simulink model "qu_sim"  (R2020a)
settings: Solver=FixedStepAuto  StartTime=0.0  StopTime=500  RelTol=1e-3
values from neighbouring files (symbols this model uses):
  n = 10    [Lab_1_kod.m]    (also in lab1.m)
undefined symbols (not defined in the file or in its folder): m
libraries: dspstat3 x1
settings Model: Creator=Bennu  LastModifiedBy=Piotr
settings DataIOCC: SaveOutput=off  SaveTime=off  ReturnWorkspaceOutputs=off
settings DebuggingCC: ArithmeticOperatorsInVariantConditions=warning
settings SFSimCC: SimUseLocalCustomCode=off  CustomCodeUndefinedFunction=UseInterfaceOnly
settings RTWCC: RTWUseLocalCustomCode=off
settings CodeAppCC: StateflowObjectComments=on

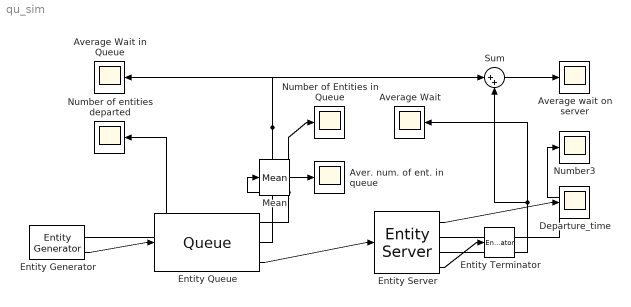
== system qu_sim ==
  Aver. num. of ent. in queue : Scope
  "Average Wait " : Scope
  Average Wait in Queue : Scope
  Average wait on server : Scope
  Departure_time : Scope
  Entity Generator : EntityGenerator  OutputPortMessageModes=n,m  TimeSource=MATLAB action  IntergenerationTimeAction=|  GenerateEntityAtSimulationStart=off  GenerateAction=|  AttributeName=Number|O_T|PriorityA  AttributeInitialValue=0|0|0  NumberEntitiesDeparted=on  EntityType=Structured  EntityTypeName=Entity
      | % Pattern: Repeating Sequence
      | persistent SEQ;
      | persistent idx;
      | if isempty(SEQ)
      |     SEQ = [12 30 29 40 12 29 14 60 84 70];
      |     %SEQ = [0 0 0 0 0 0 0 0 0 0];
      |     idx = 1;
      | end
      | if idx > numel(SEQ)
      |     dt = inf;
      | else
      |     dt = SEQ(idx);
      | end
      | idx = idx + 1;
      | % Pattern: Repeating Sequence
      | persistent SEQ;
      | persistent SEQ2;
      | persistent idx;
      | if isempty(SEQ)
      |     SEQ = [1 2 3 4 5 6 7 8 9 10];
      |     SEQ2 = [43 31 34 30 38 40 31 29 36 30];
      |     idx = 1;
      | end
      | if idx > numel(SEQ)
      |     entity.Number = inf;
      |     entity.O_T = inf;
      | else
      |     entity.Number = SEQ(idx);
      |     entity.O_T = SEQ2(idx);
      | end
      | coder.extrinsic('assignin');
      | idx = idx + 1;
      | 
      | persistent rngInit;
      | if isempty(rngInit)
      |     seed = 123483212;
      |     rng(seed);
      |     rngInit = true;
      | end
      | 
      | % Pattern: Exponential distribution
      | mu = 2;
      | entity.PriorityA = -mu * log(1 - rand());
      settings: OutputPortMap=o0,o3
  Entity Queue : Queue  InputPortMessageModes=m  OutputPortMessageModes=n,n,m  Capacity=inf  PrioritySource=PriorityA  SortingDirection=Descending  NumberEntitiesInBlock=on  AverageWait=on
      settings: OutputPortMap=o1,o2,o5
  Entity Server : EntityServer  InputPortMessageModes=m  OutputPortMessageModes=n,n,n,m  Capacity=1  ServiceTimeSource=Attribute  ServiceTimeAttributeName=O_T  ServiceTimeAction=|  NumberEntitiesDeparted=on  NumberEntitiesInBlock=on  AverageWait=on
      | % Pattern: Repeating Sequence
      | persistent SEQ;
      | persistent idx;
      | if isempty(SEQ)
      |     SEQ = [43 31 34 30 38 40 31 29 36 30];
      |     idx = 1;
      | end
      | if idx > numel(SEQ)
      |     dt = inf;
      | else
      |     dt = SEQ(idx);
      | end
      | idx = idx + 1;
      settings: OutputPortMap=o0,o1,o4,o9
  Entity Terminator : EntityTerminator  InputPortMessageModes=m  EntryAction=|
      | persistent idx;
      | coder.extrinsic('assignin');
      | persistent a;
      | if isempty(a)
      |     a = [0 0 0 0 0 0 0 0 0 0];
      |     idx = 1;
      | end
      | a(idx)=entity.Number;
      | if idx == 10
      |     assignin('base', 'inc_nr_order', a);
      | end
      | 
      | idx = idx+1;
  Mean : dspstat3/Mean  run=on  InputProcessing=Columns as channels (frame based)  reset_popup=None  directionMode=Entire input  dimension=1  roiEnable=off  roiType=Rectangles  roiPortion=Entire ROI  roiOutput=Individual statistics for each ROI  roiFlag=off  roundingMode=Floor  overflowMode=off  outputDataTypeStr=Inherit: Same as accumulator  outputMin=[]  outputMax=[]  outputLastDataTypeStr=Inherit: Same as accumulator
  Number of Entities in Queue : Scope
  Number of entities departed : Scope
  Number3 : Scope
  Sum : Sum  Inputs=|++
  wires:
  Mean/1 -> Aver. num. of ent. in queue/1
  Entity Generator/1 -> Number of entities departed/1
  Sum/1 -> Average wait on server/1
  Entity Queue/3 -> Entity Server/1
  Entity Queue/1 -> Number of Entities in Queue/1, Mean/1
  Entity Server/3 -> "Average Wait "/1, Sum/2
  Entity Server/2 -> Number3/1
  Entity Queue/2 -> Sum/1, Average Wait in Queue/1
  Entity Server/4 -> Entity Terminator/1
  Entity Generator/2 -> Entity Queue/1
  Entity Server/1 -> Departure_time/1
